simulink model "ultrasonic"  (R2016b)
settings: Solver=VariableStepAuto  StartTime=0.0  StopTime=10.0  RelTol=1e-3
values from neighbouring files (symbols this model uses):
  b = 16    [Script_controller.m]
libraries: legoev3lib x1
settings Model: Creator=karanverma  LastModifiedBy=karanverma

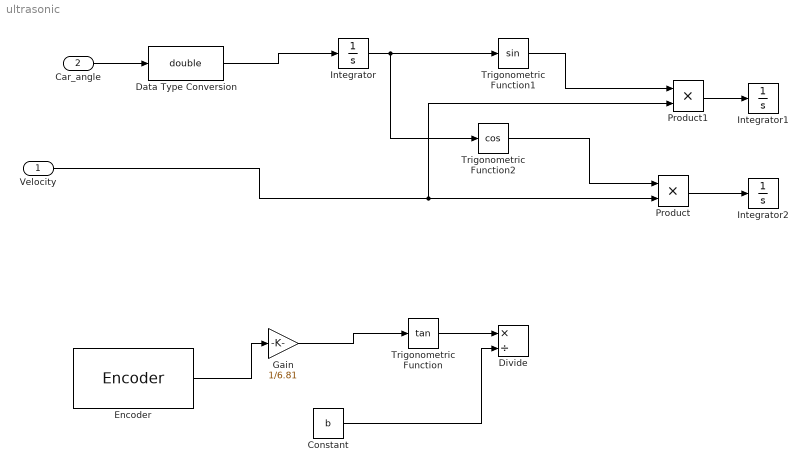
== system ultrasonic ==
  "Velocity " : Inport
  Car_angle : Inport  Port=2
  Constant : Constant  Value=b
  Data Type Conversion : DataTypeConversion  OutDataTypeStr=double
  Divide : Product  Inputs=*/
  Encoder : legoev3lib/Encoder  portNumber=A  opMode=No reset  sampleTime=0.1
  Gain : Gain  Gain=1/6.81
  Integrator : Integrator
  Integrator1 : Integrator
  Integrator2 : Integrator
  Product : Product
  Product1 : Product
  Trigonometric Function : Trigonometry  Operator=tan
  Trigonometric Function1 : Trigonometry
  Trigonometric Function2 : Trigonometry  Operator=cos
  wires:
  Car_angle/1 -> Data Type Conversion/1
  Encoder/1 -> Gain/1
  Gain/1 -> Trigonometric Function/1
  Trigonometric Function/1 -> Divide/1
  Constant/1 -> Divide/2
  Integrator/1 -> Trigonometric Function2/1, Trigonometric Function1/1
  "Velocity "/1 -> Product1/2, Product/2
  Trigonometric Function2/1 -> Product/1
  Trigonometric Function1/1 -> Product1/1
  Product/1 -> Integrator2/1
  Product1/1 -> Integrator1/1
  Data Type Conversion/1 -> Integrator/1
